simulink model "quaternion_6dof"  (R2018a)
settings: Solver=VariableStepAuto  StartTime=0.0  StopTime=3.5  RelTol=1e-3
libraries: simulink x4, aerolibutil x2, simulink_extras x2, shared6dof x1, aerolibanim x1, sharedutil x1, sharedtransform x1
settings Model: Creator=BPSSSSSPACE  LastModifiedBy=JOEYUCHECKEDTHESOURCECODE

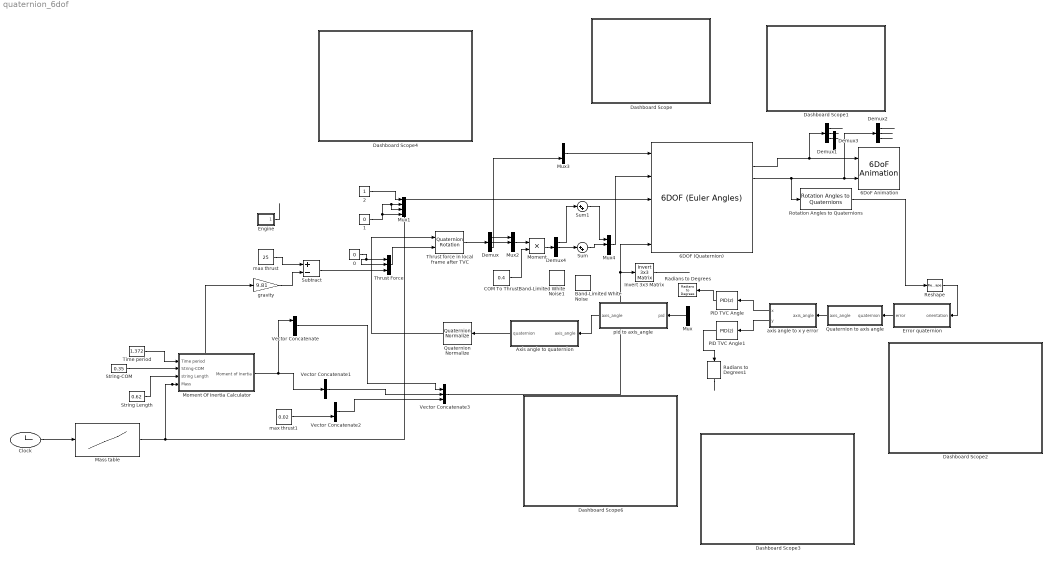
== system quaternion_6dof ==
  0 : Constant  Value=0
  1 : Constant  Value=0
  2 : Constant
  6DOF (Quaternion) : shared6dof/6DOF (Euler Angles)  units=Metric (MKS)  mtype=Custom Variable  rep=Quaternion  xme_0=[0 0 0]  Vm_0=[0 0 0]  eul_0=[0 0 0]  pm_0=[0 0 0]  mass_0=1.0  mass_e=0.5  mass_f=2.0  inertia=eye(3)  inertia_e=eye(3)  inertia_f=2*eye(3)  k_quat=1.0  vre_flag=off  abi_flag=off  aMode=0
      settings: SourceProductBaseCode=AE
  6DoF Animation : aerolibanim/6DoF Animation  u1=[0 4000 -2000 2000 -5000 -3000]  u2=0.1  u3=1.0  u4=[4000 0 -5000]  u5=Fixed position  u6=[2000 500 -3150]  u7=10  u8=on
      settings: SourceProductName=Aerospace Blockset
  Axis angle to quaternion : MATLAB Function  TreatAsAtomicUnit=on
  Band-Limited White Noise : simulink/Sources/Band-Limited White Noise  Cov=[0.01]  Ts=1  seed=[23341]
  Band-Limited White Noise1 : simulink/Sources/Band-Limited White Noise  Cov=[0.01]  Ts=1  seed=[23341]
  COM To Thrust : Constant  Value=0.4
  Clock : Clock
  Dashboard Scope : Subsystem  DialogController=hmiCreateDDGDialog  IsWebBlock=on  mask(MWDashboardBlock){webBlockId=9129ad40-3d38-4259-a345-09fc08233082, webBlockType=sdiscope, ShowInitialText=on, HMISrcModelName=quaternion_6dof}
      mask prompts: webBlockId "WebBlock Id"; webBlockType "WebBlock Type"; HMISrcModelName "Source Model"
      mask help: SimulinkHMI:dialogs:HMIScopeDialogDesc
      mask Help: helpview([docroot '/mapfiles/simulink.map'], 'hmi_scope')
      mask Display:
      | if strcmp(get_param(bdroot(gcb),'BlockDiagramType'), 'library')
      |     image([(matlabroot) '/toolbox/simulink/hmi/icons/DashboardScope.png']);
      | end
  Dashboard Scope1 : Subsystem  DialogController=hmiCreateDDGDialog  IsWebBlock=on  mask(MWDashboardBlock){webBlockId=e5edbc95-e66e-4cca-9bc8-87d3837df9bd, webBlockType=sdiscope, ShowInitialText=on, HMISrcModelName=quaternion_6dof}
      mask prompts: webBlockId "WebBlock Id"; webBlockType "WebBlock Type"; HMISrcModelName "Source Model"
      mask help: SimulinkHMI:dialogs:HMIScopeDialogDesc
      mask Help: helpview([docroot '/mapfiles/simulink.map'], 'hmi_scope')
      mask Display:
      | if strcmp(get_param(bdroot(gcb),'BlockDiagramType'), 'library')
      |     image([(matlabroot) '/toolbox/simulink/hmi/icons/DashboardScope.png']);
      | end
  Dashboard Scope2 : Subsystem  DialogController=hmiCreateDDGDialog  IsWebBlock=on  mask(MWDashboardBlock){webBlockId=8b4cce13-36b0-4b47-b7dc-7815862160cf, webBlockType=sdiscope, ShowInitialText=on, HMISrcModelName=quaternion_6dof}
      mask prompts: webBlockId "WebBlock Id"; webBlockType "WebBlock Type"; HMISrcModelName "Source Model"
      mask help: SimulinkHMI:dialogs:HMIScopeDialogDesc
      mask Help: helpview([docroot '/mapfiles/simulink.map'], 'hmi_scope')
      mask Display:
      | if strcmp(get_param(bdroot(gcb),'BlockDiagramType'), 'library')
      |     image([(matlabroot) '/toolbox/simulink/hmi/icons/DashboardScope.png']);
      | end
  Dashboard Scope3 : Subsystem  DialogController=hmiCreateDDGDialog  IsWebBlock=on  mask(MWDashboardBlock){webBlockId=268f244e-8606-4fa1-8752-6b02058021b8, webBlockType=sdiscope, ShowInitialText=on, HMISrcModelName=quaternion_6dof}
      mask prompts: webBlockId "WebBlock Id"; webBlockType "WebBlock Type"; HMISrcModelName "Source Model"
      mask help: SimulinkHMI:dialogs:HMIScopeDialogDesc
      mask Help: helpview([docroot '/mapfiles/simulink.map'], 'hmi_scope')
      mask Display:
      | if strcmp(get_param(bdroot(gcb),'BlockDiagramType'), 'library')
      |     image([(matlabroot) '/toolbox/simulink/hmi/icons/DashboardScope.png']);
      | end
  Dashboard Scope4 : Subsystem  DialogController=hmiCreateDDGDialog  IsWebBlock=on  mask(MWDashboardBlock){webBlockId=3b83e1d5-ccc4-4449-8da3-487fb1685657, webBlockType=sdiscope, ShowInitialText=on, HMISrcModelName=quaternion_6dof}
      mask prompts: webBlockId "WebBlock Id"; webBlockType "WebBlock Type"; HMISrcModelName "Source Model"
      mask help: SimulinkHMI:dialogs:HMIScopeDialogDesc
      mask Help: helpview([docroot '/mapfiles/simulink.map'], 'hmi_scope')
      mask Display:
      | if strcmp(get_param(bdroot(gcb),'BlockDiagramType'), 'library')
      |     image([(matlabroot) '/toolbox/simulink/hmi/icons/DashboardScope.png']);
      | end
  Dashboard Scope6 : Subsystem  DialogController=hmiCreateDDGDialog  IsWebBlock=on  mask(MWDashboardBlock){webBlockId=432f0317-e002-46f8-8147-c0327876a099, webBlockType=sdiscope, ShowInitialText=on, HMISrcModelName=quaternion_6dof}
      mask prompts: webBlockId "WebBlock Id"; webBlockType "WebBlock Type"; HMISrcModelName "Source Model"
      mask help: SimulinkHMI:dialogs:HMIScopeDialogDesc
      mask Help: helpview([docroot '/mapfiles/simulink.map'], 'hmi_scope')
      mask Display:
      | if strcmp(get_param(bdroot(gcb),'BlockDiagramType'), 'library')
      |     image([(matlabroot) '/toolbox/simulink/hmi/icons/DashboardScope.png']);
      | end
  Demux{,1..4} (5 alike) : Demux  Outputs=3
  Engine : Subsystem
  Error quaternion : MATLAB Function  TreatAsAtomicUnit=on
  Invert 3x3 Matrix : aerolibutil/Invert  3x3 Matrix
  Mass table : Lookup  InputValues=[0,1]  Table=[0.975,.8]  LookUpMeth=Use Input Nearest  SaturateOnIntegerOverflow=on
  Moment : Product
  Moment Of Inertia Calculator : Subsystem
  Mux : Mux  Inputs=2
  Mux1 : Mux
  Mux2 : Mux  Inputs=3
  Mux3 : Mux  Inputs=3
  Mux4 : Mux  Inputs=3
  PID TVC Angle : simulink/Continuous/PID Controller  Controller=PID  TimeDomain=Discrete-time  SampleTime=0.02  IntegratorMethod=Trapezoidal  FilterMethod=Trapezoidal  Form=Parallel  UseFilter=on  ControllerParametersSource=internal  P=0.0444910192906637  I=0.00251899563332339  D=0.170401833942346  N=91.5676010079333  InitialConditionSource=internal  InitialConditionForIntegrator=0  InitialConditionForFilter=0  ExternalReset=none  LimitOutput=on  UpperSaturationLimit=0.1745329252  LowerSaturationLimit=-0.1745329252  LinearizeAsGain=on  AntiWindupMode=none  Kb=1  TrackingMode=off  Kt=1  PParamMin=[]  PParamMax=[]  IParamMin=[]  IParamMax=[]  DParamMin=[]  DParamMax=[]  NParamMin=[]  NParamMax=[]  KbParamMin=[]  KbParamMax=[]  KtParamMin=[]  KtParamMax=[]  POutMin=[]  POutMax=[]  IOutMin=[]  IOutMax=[]  DOutMin=[]  DOutMax=[]  NOutMin=[]  NOutMax=[]  KbOutMin=[]  KbOutMax=[]  KtOutMin=[]  KtOutMax=[]  IntegratorOutMin=[]  IntegratorOutMax=[]  FilterOutMin=[]  FilterOutMax=[]  SumOutMin=[]  SumOutMax=[]  SumI1OutMin=[]  SumI1OutMax=[]  SumI2OutMin=[]  SumI2OutMax=[]  SumI3OutMin=[]  SumI3OutMax=[]  SumDOutMin=[]  SumDOutMax=[]  SaturationOutMin=[]  SaturationOutMax=[]  IntegratorContinuousStateAttributes=''  IntegratorStateMustResolveToSignalObject=off  IntegratorRTWStateStorageClass=Auto  FilterContinuousStateAttributes=''  FilterStateMustResolveToSignalObject=off  FilterRTWStateStorageClass=Auto  DifferentiatorICPrevScaledInput=0  DifferentiatorOutMin=[]  DifferentiatorOutMax=[]  FilterDiffOutCoefMin=[]  FilterDiffOutCoefMax=[]  SumDenOutMin=[]  SumDenOutMax=[]  SumNumOutMin=[]  SumNumOutMax=[]  ReciprocalOutMin=[]  ReciprocalOutMax=[]  DivideOutMin=[]  DivideOutMax=[]  TunerSelectOption=Transfer Function Based (PID Tuner App)
  PID TVC Angle1 : simulink/Continuous/PID Controller  Controller=PID  TimeDomain=Discrete-time  SampleTime=0.02  IntegratorMethod=Trapezoidal  FilterMethod=Trapezoidal  Form=Parallel  UseFilter=on  ControllerParametersSource=internal  P=0.0444910192906637  I=0.00251899563332339  D=0.170401833942346  N=91.5676010079333  InitialConditionSource=internal  InitialConditionForIntegrator=0  InitialConditionForFilter=0  ExternalReset=none  LimitOutput=on  UpperSaturationLimit=0.1745329252  LowerSaturationLimit=-0.1745329252  LinearizeAsGain=on  AntiWindupMode=none  Kb=1  TrackingMode=off  Kt=1  PParamMin=[]  PParamMax=[]  IParamMin=[]  IParamMax=[]  DParamMin=[]  DParamMax=[]  NParamMin=[]  NParamMax=[]  KbParamMin=[]  KbParamMax=[]  KtParamMin=[]  KtParamMax=[]  POutMin=[]  POutMax=[]  IOutMin=[]  IOutMax=[]  DOutMin=[]  DOutMax=[]  NOutMin=[]  NOutMax=[]  KbOutMin=[]  KbOutMax=[]  KtOutMin=[]  KtOutMax=[]  IntegratorOutMin=[]  IntegratorOutMax=[]  FilterOutMin=[]  FilterOutMax=[]  SumOutMin=[]  SumOutMax=[]  SumI1OutMin=[]  SumI1OutMax=[]  SumI2OutMin=[]  SumI2OutMax=[]  SumI3OutMin=[]  SumI3OutMax=[]  SumDOutMin=[]  SumDOutMax=[]  SaturationOutMin=[]  SaturationOutMax=[]  IntegratorContinuousStateAttributes=''  IntegratorStateMustResolveToSignalObject=off  IntegratorRTWStateStorageClass=Auto  FilterContinuousStateAttributes=''  FilterStateMustResolveToSignalObject=off  FilterRTWStateStorageClass=Auto  DifferentiatorICPrevScaledInput=0  DifferentiatorOutMin=[]  DifferentiatorOutMax=[]  FilterDiffOutCoefMin=[]  FilterDiffOutCoefMax=[]  SumDenOutMin=[]  SumDenOutMax=[]  SumNumOutMin=[]  SumNumOutMax=[]  ReciprocalOutMin=[]  ReciprocalOutMax=[]  DivideOutMin=[]  DivideOutMax=[]  TunerSelectOption=Transfer Function Based (PID Tuner App)
  Quaternion Normalize : sharedutil/Quaternion Normalize  aMode=aMode
      settings: SourceProductName=Aerospace Blockset  SourceProductBaseCode=AE
  Quaternion to axis angle : MATLAB Function  TreatAsAtomicUnit=on
  Radians to Degrees : simulink_extras/Transformations/Radians to Degrees
  Radians to Degrees1 : simulink_extras/Transformations/Radians to Degrees
  Reshape : Reshape  OutputDimensionality=Row vector (2-D)
  Rotation Angles to Quaternions : sharedtransform/Rotation Angles to Quaternions  rotationOrder=XYZ  aMode=aMode
      settings: SourceProductName=Aerospace Blockset  SourceProductBaseCode=AE
  String Length : Constant  Value=0.62
  String-COM : Constant  Value=0.35
  Subtract : Sum  Inputs=+-
  Sum : Sum  Inputs=|++
  Sum1 : Sum  Inputs=|++
  Thrust Force : Mux  Inputs=3
  Thrust force in local frame after TVC : aerolibutil/Quaternion Rotation
  Time period : Constant  Value=1.372
  Vector Concatenate : Concatenate  NumInputs=3
  Vector Concatenate1 : Concatenate  NumInputs=3
  Vector Concatenate2 : Concatenate  NumInputs=3
  Vector Concatenate3 : Concatenate  NumInputs=3  Mode=Multidimensional array  ConcatenateDimension=2
  axis angle to x y error : MATLAB Function  TreatAsAtomicUnit=on
  gravity : Gain  Gain=9.81
  max thrust : Constant  Value=25
  max thrust1 : Constant  Value=0.02
  pid to axis_angle : MATLAB Function  TreatAsAtomicUnit=on
  wires:
  Thrust force in local frame after TVC/1 -> Demux/1
  Demux/1 -> Mux2/1
  Demux/2 -> Mux2/2
  Mux2/1 -> Moment/1
  COM To Thrust/1 -> Moment/2
  Thrust Force/1 -> Thrust force in local frame after TVC/2
  6DOF (Quaternion)/3 -> Rotation Angles to Quaternions/1, Demux2/1, 6DoF Animation/2
  6DOF (Quaternion)/2 -> Demux1/1, 6DoF Animation/1
  Moment Of Inertia Calculator/1(Moment of Inertia) -> Vector Concatenate/1, Vector Concatenate1/2
  0/1 -> Thrust Force/2, Thrust Force/1
  Time period/1 -> Moment Of Inertia Calculator/1(Time period)
  String Length/1 -> Moment Of Inertia Calculator/3(string Length)
  Clock/1 -> Mass table/1
  Mass table/1 -> 6DOF (Quaternion)/3, gravity/1, Moment Of Inertia Calculator/4(Mass)
  String-COM/1 -> Moment Of Inertia Calculator/2(String-COM)
  Demux/3 -> Mux3/3
  max thrust1/1 -> Vector Concatenate2/3
  Vector Concatenate2/1 -> Vector Concatenate3/3
  Vector Concatenate1/1 -> Vector Concatenate3/2
  Vector Concatenate/1 -> Vector Concatenate3/1
  Invert 3x3 Matrix/1 -> ?
  Vector Concatenate3/1 -> 6DOF (Quaternion)/5, Invert 3x3 Matrix/1
  2/1 -> Mux1/1
  1/1 -> Mux1/4, Mux1/3, Mux1/2
  Mux3/1 -> 6DOF (Quaternion)/1
  Demux1/1 -> ?
  Demux1/2 -> ?
  Demux1/3 -> ?
  Demux2/3 -> ?
  Demux2/2 -> ?
  Demux2/1 -> ?
  Engine/1(Thrust) -> ?
  Subtract/1 -> Thrust Force/3
  gravity/1 -> Subtract/2
  Rotation Angles to Quaternions/1 -> Reshape/1
  Reshape/1 -> Error quaternion/1(orientation)
  Error quaternion/1(error) -> Quaternion to axis angle/1(quaternion)
  pid to axis_angle/1(axis_angle) -> Axis angle to quaternion/1(axis_angle)
  max thrust/1 -> Subtract/1
  Moment/1 -> Demux4/1
  Quaternion to axis angle/1(axis_angle) -> axis angle to x y error/1(axis_angle)
  axis angle to x y error/1(x) -> PID TVC Angle/1
  axis angle to x y error/2(y) -> PID TVC Angle1/1
  Mux/1 -> pid to axis_angle/1(pid)
  Mux4/1 -> 6DOF (Quaternion)/2
  Sum/1 -> Mux4/2
  Demux4/2 -> Sum/1
  Demux4/1 -> Sum1/1
  Sum1/1 -> Mux4/1
  Radians to Degrees1/1 -> ?
  PID TVC Angle1/1 -> Radians to Degrees1/1
  PID TVC Angle/1 -> Radians to Degrees/1
  Axis angle to quaternion/1(quaternion) -> Quaternion Normalize/1
  Quaternion Normalize/1 -> Thrust force in local frame after TVC/1

== system quaternion_6dof/Dashboard Scope ==

== system quaternion_6dof/Dashboard Scope1 ==

== system quaternion_6dof/Dashboard Scope2 ==

== system quaternion_6dof/Dashboard Scope3 ==

== system quaternion_6dof/Dashboard Scope4 ==

== system quaternion_6dof/Dashboard Scope6 ==

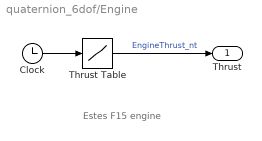
== system quaternion_6dof/Engine ==
  note: Estes F15 engine
  Clock : Clock
  Thrust Table : Lookup  InputValues=|  Table=[0,12.5,25,16.5,15.25,15,14.5,14.5,14.25,14,13,13,0]  LookUpMeth=Interpolation-Use End Values  SaturateOnIntegerOverflow=on
      | [0,
      | 0.25,
      | 0.5,
      | 0.75,
      | 1,
      | 1.25,
      | 1.5,
      | 2,
      | 2.25,
      | 2.5,
      | 3,
      | 3.25,
      | 3.5]
  Thrust : Outport
  wires:
  Clock/1 -> Thrust Table/1
  Thrust Table/1 -> Thrust/1  "EngineThrust_nt"

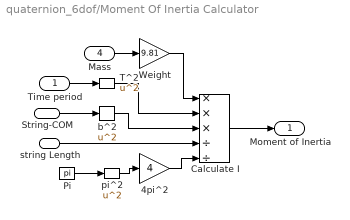
== system quaternion_6dof/Moment Of Inertia Calculator ==
  Time period : Inport
  String-COM : Inport  Port=2
  string Length : Inport  Port=3
  Mass : Inport  Port=4
  4pi^2 : Gain  Gain=4
  Calculate I : Product  Inputs=***//
  Pi : Constant  Value=pi
  T^2 : Math  Operator=square  SaturateOnIntegerOverflow=on
  Weight : Gain  Gain=9.81
  b^2 : Math  Operator=square  SaturateOnIntegerOverflow=on
  pi^2 : Math  Operator=square  SaturateOnIntegerOverflow=on
  Moment of Inertia : Outport
  wires:
  Time period/1 -> T^2/1
  Calculate I/1 -> Moment of Inertia/1
  string Length/1 -> Calculate I/4
  Mass/1 -> Weight/1
  Weight/1 -> Calculate I/1
  pi^2/1 -> 4pi^2/1
  b^2/1 -> Calculate I/3
  T^2/1 -> Calculate I/2
  String-COM/1 -> b^2/1
  Pi/1 -> pi^2/1
  4pi^2/1 -> Calculate I/5

== matlab function quaternion_6dof/axis angle to x y error ==
  settings: updateMethod=DISCRETE
  data: axis_angle input; x output; y output
function [x,y] = fcn(axis_angle)

y= axis_angle(1) * axis_angle(2);
x= axis_angle(1) * axis_angle(3);

== matlab function quaternion_6dof/Error quaternion ==
  data: orientation input; error output
function error = fcn(orientation)

if abs(orientation(1)) ~= 1
    theta = acos(orientation(1));
    x = atan(tan(theta) * orientation(4)/sin(theta));
    roll = [cos(x), 0, 0,sin(x)];
    error = quatmultiply(quatinv(orientation), roll);
    t = acos(error(1));
    if t < 0
        error(1) = cos(pi - t);
    end
    %if t < -pi/2
        %error(1) = cos(t + pi); %if more than -180 degree rotation add 360 degrees to angle, only pi as q0 is divided by 2
    %elseif t > pi/2
        %error(1) = cos(t - pi); %if more than 180 degree rotation subtract 360 degrees to angle, only pi as q0 is divided by 2
    %end
else
    error = [1 0 0 0];
end

== matlab function quaternion_6dof/Quaternion to axis angle ==
  settings: updateMethod=DISCRETE
  data: quaternion input; axis_angle output
function axis_angle = fcn(quaternion)

persistent previous_axis_vector;

if abs(quaternion(1)) == 1
    angle = 0; %if 0 degree rotation dont divide by 0 http://www.euclideanspace.com/maths/geometry/rotations/conversions/quaternionToAngle/ 
else
    s = (1-quaternion(1)^2)^0.5;
    previous_axis_vector = [quaternion(2) quaternion(3) quaternion(4)] / s;
    angle = 2 * acos(quaternion(1));
end

if isempty(previous_axis_vector)
    previous_axis_vector = [1 0 0];
end

axis_angle = [angle previous_axis_vector];

== matlab function quaternion_6dof/Axis angle to quaternion ==
  data: axis_angle input; quaternion output
function quaternion = fcn(axis_angle)

angle = axis_angle(1)/2;
sine = sin(angle);
quaternion = [cos(angle); sine * axis_angle(2); sine * axis_angle(3); sine * axis_angle(4)];

== matlab function quaternion_6dof/pid to axis_angle ==
  settings: updateMethod=DISCRETE
  data: pid input; axis_angle output
function axis_angle = fcn(pid)

angle = norm(pid);
if angle == 0
    v = [1 0];
else
    v = [pid(1)/angle pid(2)/angle];
end
axis_angle = [angle v 0];
